simulink model "PD"  (R2015a)
settings: Solver=ode45  StartTime=0.0  StopTime=100  RelTol=1e-3  AbsTol=1e-6
libraries: cstblocks x6
settings Model: Creator=ANILKUMAR  LastModifiedBy=dj

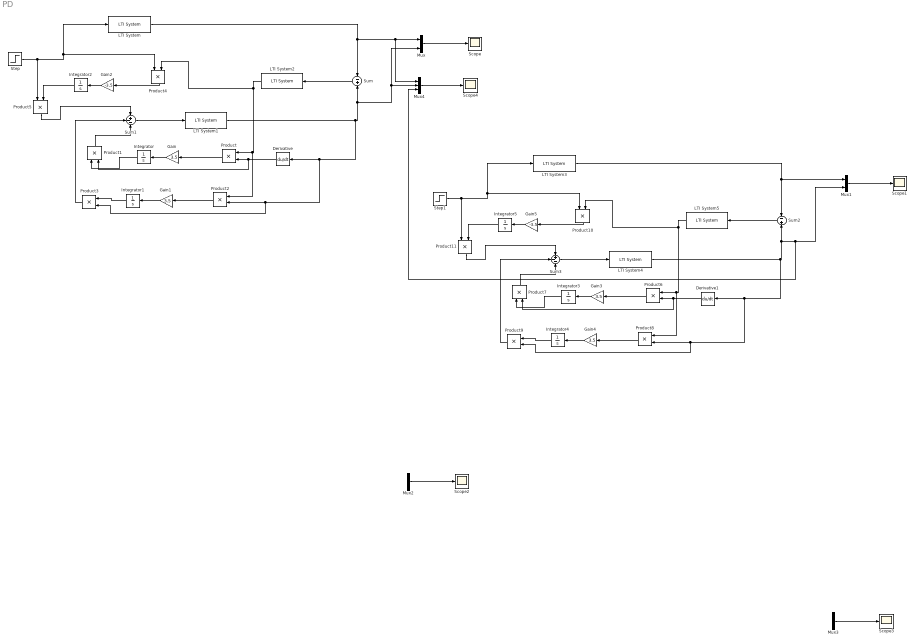
== system PD ==
  Derivative : Derivative
  Derivative1 : Derivative
  Gain{,1,3..4} (4 alike) : Gain  Gain=3.5
  Gain2 : Gain  Gain=-3.5
  Gain5 : Gain  Gain=-3.5
  Integrator{,1..5} (6 alike) : Integrator
  LTI System : cstblocks/LTI System  sys=tf(25,[1 6 25])  IC=[]
  LTI System1 : cstblocks/LTI System  sys=tf(.3,[1 .3 .6])  IC=[]
  LTI System2 : cstblocks/LTI System  sys=tf(1,[1 6 25])  IC=[]
  LTI System3 : cstblocks/LTI System  sys=tf(25,[1 6 25])  IC=[]
  LTI System4 : cstblocks/LTI System  sys=tf(.3,[1 .6 .10])  IC=[]
  LTI System5 : cstblocks/LTI System  sys=tf(1,[1 6 25])  IC=[]
  Mux{,1..3} (4 alike) : Mux  Inputs=2
  Mux4 : Mux  Inputs=3
  Product{,1..11} (12 alike) : Product
  Scope{,1..4} (5 alike) : Scope
      Scope2 settings: SaveName=ScopeData2
      Scope3 settings: SaveName=ScopeData3
      Scope4 settings: SaveName=ScopeData4
  Step : Step  SampleTime=0
  Step1 : Step  SampleTime=0
  Sum : Sum  Inputs=-+
  Sum1 : Sum  Inputs=+--
  Sum2 : Sum  Inputs=-+
  Sum3 : Sum  Inputs=+--
  wires:
  Step/1 -> Product5/1, LTI System/1, Product4/1
  LTI System/1 -> Mux4/1, Mux/1, Sum/1
  LTI System1/1 -> Product3/2, Product2/2, Derivative/1, Mux4/2, Mux/2, Sum/2
  Derivative/1 -> Product1/2, Product/2
  Sum/1 -> LTI System2/1
  LTI System2/1 -> Product4/2, Product2/1, Product/1
  Product/1 -> Gain/1
  Gain/1 -> Integrator/1
  Integrator/1 -> Product1/1
  Sum1/1 -> LTI System1/1
  Product1/1 -> Sum1/3
  Product2/1 -> Gain1/1
  Gain1/1 -> Integrator1/1
  Integrator1/1 -> Product3/1
  Product3/1 -> Sum1/2
  Product4/1 -> Gain2/1
  Gain2/1 -> Integrator2/1
  Integrator2/1 -> Product5/2
  Product5/1 -> Sum1/1
  Mux/1 -> Scope/1
  Mux2/1 -> Scope2/1
  Step1/1 -> Product11/1, LTI System3/1, Product10/1
  LTI System3/1 -> Mux1/1, Sum2/1
  Derivative1/1 -> Product7/2, Product6/2
  Sum2/1 -> LTI System5/1
  LTI System5/1 -> Product10/2, Product8/1, Product6/1
  Product6/1 -> Gain3/1
  Gain3/1 -> Integrator3/1
  Integrator3/1 -> Product7/1
  Sum3/1 -> LTI System4/1
  Product7/1 -> Sum3/3
  Product8/1 -> Gain4/1
  Gain4/1 -> Integrator4/1
  Integrator4/1 -> Product9/1
  Product9/1 -> Sum3/2
  Product10/1 -> Gain5/1
  Gain5/1 -> Integrator5/1
  Integrator5/1 -> Product11/2
  Product11/1 -> Sum3/1
  Mux1/1 -> Scope1/1
  Mux3/1 -> Scope3/1
  LTI System4/1 -> Product9/2, Product8/2, Derivative1/1, Mux4/3, Mux1/2, Sum2/2
  Mux4/1 -> Scope4/1
